simulink model "vehicle_suspension"  (R2016a)
settings: Solver=VariableStepAuto  SolverMode=SingleTasking  StartTime=0.0  StopTime=10.0  RelTol=1e-3
values from neighbouring files (symbols this model uses):
  Vmass = 2000    [vehicle_suspension_data.mat]
  wheeltrack = 1.5    [vehicle_suspension_data.mat]
  x_dist_pass1 = 0.6    [vehicle_suspension_data.mat]
  x_dist_pass2 = 1.1    [vehicle_suspension_data.mat]
  x_dist_pass3 = 0.6    [vehicle_suspension_data.mat]
  x_dist_pass4 = 1.1    [vehicle_suspension_data.mat]
  y_dist_pass1 = 1.4    [vehicle_suspension_data.mat]
  y_dist_pass2 = 1.4    [vehicle_suspension_data.mat]
  y_dist_pass3 = 2.2    [vehicle_suspension_data.mat]
  y_dist_pass4 = 2.2    [vehicle_suspension_data.mat]
settings Model: Creator=ADYPU-LAP-3  LastModifiedBy=AkashG_v13
settings DataIOCC: ReturnWorkspaceOutputs=on
settings DebuggingCC: SFUnexpectedBacktrackingDiag=error  SFNoUnconditionalDefaultTransitionDiag=error
settings SFSimCC: SimUseLocalCustomCode=on
settings RTWCC: RTWUseLocalCustomCode=on
settings GRTTargetCC: TargetLangStandard=C99 (ISO)  GeneratePreprocessorConditionals=Use local settings
settings ConfigComp: CovMetricSettings=dwe  CovHtmlReporting=off  CovSaveCumulativeToWorkspaceVar=off  CovSaveSingleToWorkspaceVar=off  CovExternalEMLEnable=on

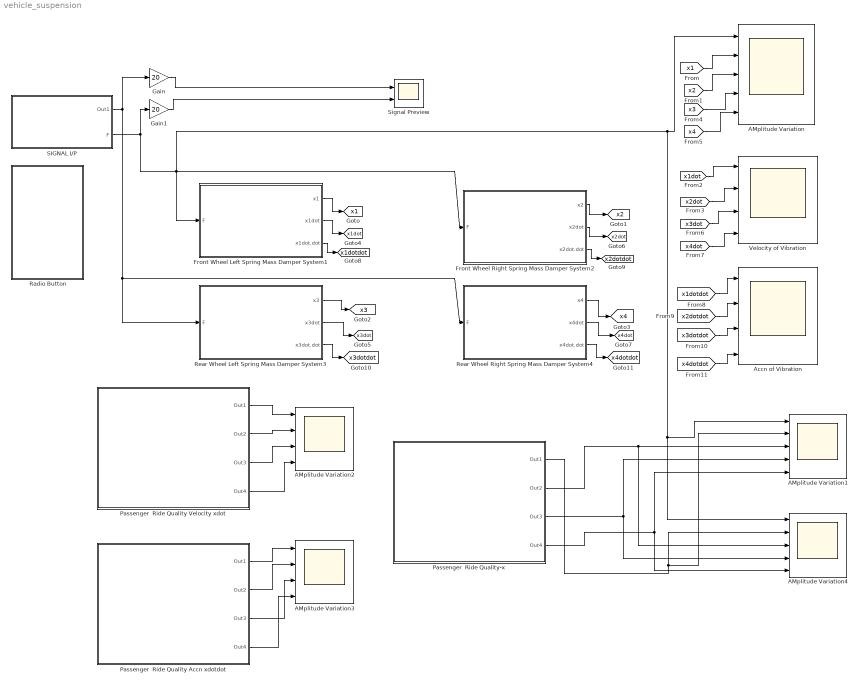
== system vehicle_suspension ==
  AMplitude Variation : Scope  NumInputPorts=5
  AMplitude Variation1 : Scope  NumInputPorts=5
  AMplitude Variation2 : Scope  NumInputPorts=4
  AMplitude Variation3 : Scope  NumInputPorts=4
  AMplitude Variation4 : Scope  NumInputPorts=5
  Accn of Vibration : Scope  NumInputPorts=4
  Front Wheel Left Spring Mass Damper System1 : Subsystem
  Front Wheel Right Spring Mass Damper System2 : Subsystem
  Gain : Gain  Gain=20
  Gain1 : Gain  Gain=20
  Passenger  Ride Quality Accn xdotdot : Subsystem
  Passenger  Ride Quality Velocity xdot : Subsystem
  Passenger  Ride Quality-x : Subsystem
  Radio Button : Subsystem  Description=Replaced Block  mask(Replaced Block){}
      mask help: This block has been replaced with an empty subsystem because it used functionality that is unavailable in Simulink R2016a.
      mask Display: fprintf('Replaced: %s\n','Dashboard Widget')
  Rear Wheel Left Spring Mass Damper System3 : Subsystem
  Rear Wheel Right Spring Mass Damper System4 : Subsystem
  SIGNAL I/P : Subsystem
  Signal Preview : Scope  NumInputPorts=2
  Velocity of Vibration : Scope  NumInputPorts=4
  tag scope: x1=global, x1dot=global, x1dotdot=global, x2=global, x2dot=global, x2dotdot=global, x3=global, x3dot=global, x3dotdot=global, x4=global, x4dot=global, x4dotdot=global
  wires:
  Front Wheel Left Spring Mass Damper System1/1(x1) -> [x1]
  Front Wheel Right Spring Mass Damper System2/1(x2) -> [x2]
  [x1] -> AMplitude Variation/2
  [x2] -> AMplitude Variation/3
  Rear Wheel Left Spring Mass Damper System3/1(x3) -> [x3]
  [x3] -> AMplitude Variation/4
  [x4] -> AMplitude Variation/5
  Rear Wheel Right Spring Mass Damper System4/1(x4) -> [x4]
  Passenger  Ride Quality-x/1(Out1) -> AMplitude Variation4/2, AMplitude Variation1/2
  Passenger  Ride Quality-x/3(Out3) -> AMplitude Variation1/4, AMplitude Variation4/4
  Passenger  Ride Quality-x/4(Out4) -> AMplitude Variation1/5, AMplitude Variation4/5
  Passenger  Ride Quality Velocity xdot/1(Out1) -> AMplitude Variation2/1
  Passenger  Ride Quality Velocity xdot/2(Out2) -> AMplitude Variation2/2
  Passenger  Ride Quality Velocity xdot/3(Out3) -> AMplitude Variation2/3
  Passenger  Ride Quality Velocity xdot/4(Out4) -> AMplitude Variation2/4
  Passenger  Ride Quality Accn xdotdot/1(Out1) -> AMplitude Variation3/1
  Passenger  Ride Quality Accn xdotdot/2(Out2) -> AMplitude Variation3/2
  Passenger  Ride Quality Accn xdotdot/3(Out3) -> AMplitude Variation3/3
  Passenger  Ride Quality Accn xdotdot/4(Out4) -> AMplitude Variation3/4
  Front Wheel Left Spring Mass Damper System1/2(x1dot) -> [x1dot]
  [x1dot] -> Velocity of Vibration/1
  Front Wheel Right Spring Mass Damper System2/2(x2dot) -> [x2dot]
  [x2dot] -> Velocity of Vibration/2
  Rear Wheel Left Spring Mass Damper System3/2(x3dot) -> [x3dot]
  [x3dot] -> Velocity of Vibration/3
  [x4dot] -> Velocity of Vibration/4
  Front Wheel Left Spring Mass Damper System1/3(x1dot.dot) -> [x1dotdot]
  Front Wheel Right Spring Mass Damper System2/3(x2dot.dot) -> [x2dotdot]
  Rear Wheel Left Spring Mass Damper System3/3(x3dot.dot) -> [x3dotdot]
  Rear Wheel Right Spring Mass Damper System4/2(x4dot) -> [x4dot]
  Rear Wheel Right Spring Mass Damper System4/3(x4dot.dot) -> [x4dotdot]
  [x1dotdot] -> Accn of Vibration/1
  [x2dotdot] -> Accn of Vibration/2
  [x3dotdot] -> Accn of Vibration/3
  [x4dotdot] -> Accn of Vibration/4
  Gain/1 -> Signal Preview/1
  Gain1/1 -> Signal Preview/2
  Passenger  Ride Quality-x/2(Out2) -> AMplitude Variation4/3, AMplitude Variation1/3
  SIGNAL I/P/2(F) -> Gain1/1, Front Wheel Left Spring Mass Damper System1/1(F), Front Wheel Right Spring Mass Damper System2/1(F), AMplitude Variation4/1, AMplitude Variation1/1, AMplitude Variation/1
  SIGNAL I/P/1(Out1) -> Rear Wheel Right Spring Mass Damper System4/1(F), Rear Wheel Left Spring Mass Damper System3/1(F), Gain/1

== system vehicle_suspension/Front Wheel Left Spring Mass Damper System1 ==
  F : Inport
  Add : Sum  Inputs=+---
  C-damping Coefficient : Gain  Gain=0.2
  Integrator : Integrator
  Integrator1 : Integrator
  Integrator2 : Integrator
  Mass-M1 : Gain  Gain=Vmass*(1.6/4)*0.5
  Spring Stiffness -K1 : Gain  Gain=2
  Spring Stifness K2 : Gain  Gain=5
  x1 : Outport
  x1dot : Outport  Port=2
  x1dot.dot : Outport  Port=3
  wires:
  C-damping Coefficient/1 -> Add/4  "C dx/dt"
  Integrator1/1 -> C-damping Coefficient/1, Integrator/1
  Spring Stiffness -K1/1 -> Add/2  "K1x"
  Integrator/1 -> x1/1, Spring Stifness K2/1, Spring Stiffness -K1/1  "x"
  Mass-M1/1 -> Integrator1/1  "M dx2/dt2"
  Spring Stifness K2/1 -> Add/3  "K2x"
  Add/1 -> Integrator2/1, x1dot.dot/1, Mass-M1/1  "d2x/dt2"
  F/1 -> Add/1
  Integrator2/1 -> x1dot/1

== system vehicle_suspension/Front Wheel Right Spring Mass Damper System2 ==
  F : Inport
  Add : Sum  Inputs=+---
  C-damping Coefficient : Gain  Gain=0.2
  Integrator : Integrator
  Integrator1 : Integrator
  Integrator2 : Integrator
  Mass-M1 : Gain  Gain=Vmass*(1.6/4)*0.5
  Spring Stiffness -K1 : Gain  Gain=2
  Spring Stifness K2 : Gain  Gain=5
  x2 : Outport
  x2dot : Outport  Port=2
  x2dot.dot : Outport  Port=3
  wires:
  Integrator2/1 -> x2dot/1
  F/1 -> Add/1
  Add/1 -> Mass-M1/1, x2dot.dot/1, Integrator2/1  "d2x/dt2"
  Spring Stifness K2/1 -> Add/3  "K2x"
  Mass-M1/1 -> Integrator1/1  "M dx2/dt2"
  Integrator/1 -> Spring Stiffness -K1/1, Spring Stifness K2/1, x2/1  "x2"
  Spring Stiffness -K1/1 -> Add/2  "K1x"
  Integrator1/1 -> Integrator/1, C-damping Coefficient/1
  C-damping Coefficient/1 -> Add/4  "C dx/dt"

== system vehicle_suspension/Passenger  Ride Quality Accn xdotdot ==
  Passenger 1 Ride Eval  x1 : Subsystem
  Passenger 2 Ride Eval  x2 : Subsystem
  Passenger 3 Ride Eval  x3 : Subsystem
  Passenger 4 Ride Eval  x4 : Subsystem
  Out1 : Outport
  Out2 : Outport  Port=2
  Out3 : Outport  Port=3
  Out4 : Outport  Port=4
  wires:
  Passenger 2 Ride Eval  x2/1(Out1) -> Out2/1
  Passenger 3 Ride Eval  x3/1(Out1) -> Out3/1
  Passenger 4 Ride Eval  x4/1(Out1) -> Out4/1
  Passenger 1 Ride Eval  x1/1(Out1) -> Out1/1

== system vehicle_suspension/Passenger  Ride Quality Velocity xdot ==
  Passenger 1 Ride Eval  x1 : Subsystem
  Passenger 2 Ride Eval  x2 : Subsystem
  Passenger 3 Ride Eval  x3 : Subsystem
  Passenger 4 Ride Eval  x4 : Subsystem
  Out1 : Outport
  Out2 : Outport  Port=2
  Out3 : Outport  Port=3
  Out4 : Outport  Port=4
  wires:
  Passenger 1 Ride Eval  x1/1(Out1) -> Out1/1
  Passenger 4 Ride Eval  x4/1(Out1) -> Out4/1
  Passenger 3 Ride Eval  x3/1(Out1) -> Out3/1
  Passenger 2 Ride Eval  x2/1(Out1) -> Out2/1

== system vehicle_suspension/Passenger  Ride Quality-x ==
  Passenger 1 Ride Eval  x1 : Subsystem
  Passenger 2 Ride Eval  x2 : Subsystem
  Passenger 3 Ride Eval  x3 : Subsystem
  Passenger 4 Ride Eval  x4 : Subsystem
  Out1 : Outport
  Out2 : Outport  Port=2
  Out3 : Outport  Port=3
  Out4 : Outport  Port=4
  wires:
  Passenger 2 Ride Eval  x2/1(Out1) -> Out2/1
  Passenger 3 Ride Eval  x3/1(Out1) -> Out3/1
  Passenger 4 Ride Eval  x4/1(Out1) -> Out4/1
  Passenger 1 Ride Eval  x1/1(Out1) -> Out1/1

== system vehicle_suspension/Radio Button ==

== system vehicle_suspension/Rear Wheel Left Spring Mass Damper System3 ==
  F : Inport
  Add : Sum  Inputs=+---
  C-damping Coefficient : Gain  Gain=0.2
  Integrator : Integrator
  Integrator1 : Integrator
  Integrator2 : Integrator
  Mass-M1 : Gain  Gain=Vmass*(1.6/4)*0.5
  Spring Stiffness -K1 : Gain  Gain=2
  Spring Stifness K2 : Gain  Gain=5
  x3 : Outport
  x3dot : Outport  Port=2
  x3dot.dot : Outport  Port=3
  wires:
  C-damping Coefficient/1 -> Add/4  "C dx/dt"
  Integrator1/1 -> C-damping Coefficient/1, Integrator/1
  Spring Stiffness -K1/1 -> Add/2  "K1x"
  Integrator/1 -> x3/1, Spring Stifness K2/1, Spring Stiffness -K1/1  "x3"
  Mass-M1/1 -> Integrator1/1  "M dx2/dt2"
  Spring Stifness K2/1 -> Add/3  "K2x"
  Add/1 -> Integrator2/1, x3dot.dot/1, Mass-M1/1  "d2x/dt2"
  F/1 -> Add/1
  Integrator2/1 -> x3dot/1

== system vehicle_suspension/Rear Wheel Right Spring Mass Damper System4 ==
  F : Inport
  Add : Sum  Inputs=+---
  C-damping Coefficient : Gain  Gain=0.2
  Integrator : Integrator
  Integrator1 : Integrator
  Integrator2 : Integrator
  Mass-M1 : Gain  Gain=Vmass*(1.6/4)*0.5
  Spring Stiffness -K1 : Gain  Gain=2
  Spring Stifness K2 : Gain  Gain=5
  x4 : Outport
  x4dot : Outport  Port=2
  x4dot.dot : Outport  Port=3
  wires:
  Integrator2/1 -> x4dot/1
  F/1 -> Add/1
  Add/1 -> Mass-M1/1, x4dot.dot/1, Integrator2/1  "d2x/dt2"
  Spring Stifness K2/1 -> Add/3  "K2x"
  Mass-M1/1 -> Integrator1/1  "M dx2/dt2"
  Integrator/1 -> Spring Stiffness -K1/1, Spring Stifness K2/1, x4/1  "x4"
  Spring Stiffness -K1/1 -> Add/2  "K1x"
  Integrator1/1 -> Integrator/1, C-damping Coefficient/1
  C-damping Coefficient/1 -> Add/4  "C dx/dt"

== system vehicle_suspension/SIGNAL I//P ==
  " " : Trigonometry  Operator=cos
  Add : Sum  Inputs=+-
  Clock : Clock
      settings: Decimation=20
  Constant1 : Constant  Value=2
  Constant2 : Constant  Value=2
  Product : Product
  Product1 : Product
  Sin : Trigonometry  Operator=cos
  Out1 : Outport
  F : Outport  Port=2
  wires:
  Constant1/1 -> Product1/1, Product/1
  Constant2/1 -> Add/2
  Add/1 -> " "/1
  " "/1 -> F/1  "F"
  Product1/1 -> Add/1
  Product/1 -> Sin/1
  Clock/1 -> Product1/2, Product/2
  Sin/1 -> Out1/1

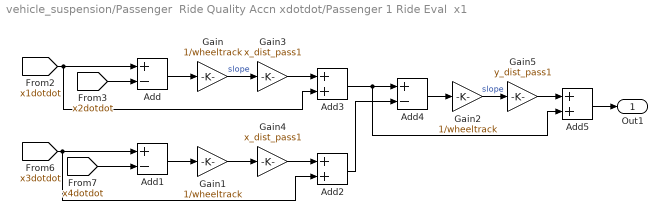
== system vehicle_suspension/Passenger  Ride Quality Accn xdotdot/Passenger 1 Ride Eval  x1 ==
  Add : Sum  Inputs=+-
  Add1 : Sum  Inputs=+-
  Add2 : Sum
  Add3 : Sum
  Add4 : Sum  Inputs=+-
  Add5 : Sum
  Gain : Gain  Gain=1/wheeltrack
  Gain1 : Gain  Gain=1/wheeltrack
  Gain2 : Gain  Gain=1/wheeltrack
  Gain3 : Gain  Gain=x_dist_pass1
  Gain4 : Gain  Gain=x_dist_pass1
  Gain5 : Gain  Gain=y_dist_pass1
  Out1 : Outport
  wires:
  Gain1/1 -> Gain4/1
  [x2dotdot] -> Add/2
  Gain2/1 -> Gain5/1  "slope"
  Gain/1 -> Gain3/1  "slope"
  [x4dotdot] -> Add1/2
  Add1/1 -> Gain1/1
  [x1dotdot] -> Add3/2, Add/1
  Add/1 -> Gain/1
  Gain3/1 -> Add3/1
  Gain4/1 -> Add2/1
  [x3dotdot] -> Add2/2, Add1/1
  Add3/1 -> Add5/2, Add4/1
  Add2/1 -> Add4/2
  Add4/1 -> Gain2/1
  Gain5/1 -> Add5/1
  Add5/1 -> Out1/1

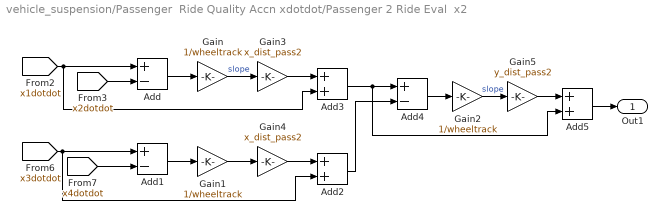
== system vehicle_suspension/Passenger  Ride Quality Accn xdotdot/Passenger 2 Ride Eval  x2 ==
  Add : Sum  Inputs=+-
  Add1 : Sum  Inputs=+-
  Add2 : Sum
  Add3 : Sum
  Add4 : Sum  Inputs=+-
  Add5 : Sum
  Gain : Gain  Gain=1/wheeltrack
  Gain1 : Gain  Gain=1/wheeltrack
  Gain2 : Gain  Gain=1/wheeltrack
  Gain3 : Gain  Gain=x_dist_pass2
  Gain4 : Gain  Gain=x_dist_pass2
  Gain5 : Gain  Gain=y_dist_pass2
  Out1 : Outport
  wires:
  Add5/1 -> Out1/1
  Gain5/1 -> Add5/1
  Add4/1 -> Gain2/1
  Add2/1 -> Add4/2
  Add3/1 -> Add4/1, Add5/2
  [x3dotdot] -> Add1/1, Add2/2
  Gain4/1 -> Add2/1
  Gain3/1 -> Add3/1
  Add/1 -> Gain/1
  [x1dotdot] -> Add/1, Add3/2
  Add1/1 -> Gain1/1
  [x4dotdot] -> Add1/2
  Gain/1 -> Gain3/1  "slope"
  Gain2/1 -> Gain5/1  "slope"
  [x2dotdot] -> Add/2
  Gain1/1 -> Gain4/1

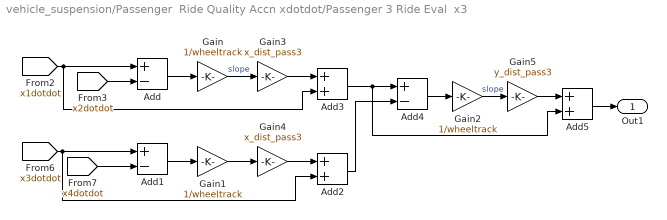
== system vehicle_suspension/Passenger  Ride Quality Accn xdotdot/Passenger 3 Ride Eval  x3 ==
  Add : Sum  Inputs=+-
  Add1 : Sum  Inputs=+-
  Add2 : Sum
  Add3 : Sum
  Add4 : Sum  Inputs=+-
  Add5 : Sum
  Gain : Gain  Gain=1/wheeltrack
  Gain1 : Gain  Gain=1/wheeltrack
  Gain2 : Gain  Gain=1/wheeltrack
  Gain3 : Gain  Gain=x_dist_pass3
  Gain4 : Gain  Gain=x_dist_pass3
  Gain5 : Gain  Gain=y_dist_pass3
  Out1 : Outport
  wires:
  Gain1/1 -> Gain4/1
  [x2dotdot] -> Add/2
  Gain2/1 -> Gain5/1  "slope"
  Gain/1 -> Gain3/1  "slope"
  [x4dotdot] -> Add1/2
  Add1/1 -> Gain1/1
  [x1dotdot] -> Add3/2, Add/1
  Add/1 -> Gain/1
  Gain3/1 -> Add3/1
  Gain4/1 -> Add2/1
  [x3dotdot] -> Add2/2, Add1/1
  Add3/1 -> Add5/2, Add4/1
  Add2/1 -> Add4/2
  Add4/1 -> Gain2/1
  Gain5/1 -> Add5/1
  Add5/1 -> Out1/1

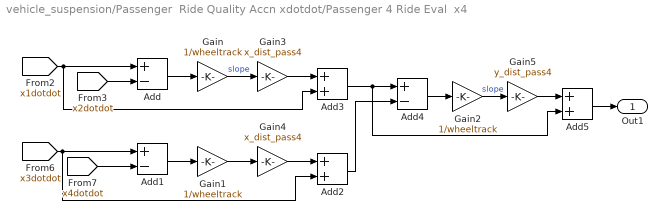
== system vehicle_suspension/Passenger  Ride Quality Accn xdotdot/Passenger 4 Ride Eval  x4 ==
  Add : Sum  Inputs=+-
  Add1 : Sum  Inputs=+-
  Add2 : Sum
  Add3 : Sum
  Add4 : Sum  Inputs=+-
  Add5 : Sum
  Gain : Gain  Gain=1/wheeltrack
  Gain1 : Gain  Gain=1/wheeltrack
  Gain2 : Gain  Gain=1/wheeltrack
  Gain3 : Gain  Gain=x_dist_pass4
  Gain4 : Gain  Gain=x_dist_pass4
  Gain5 : Gain  Gain=y_dist_pass4
  Out1 : Outport
  wires:
  Add5/1 -> Out1/1
  Gain5/1 -> Add5/1
  Add4/1 -> Gain2/1
  Add2/1 -> Add4/2
  Add3/1 -> Add4/1, Add5/2
  [x3dotdot] -> Add1/1, Add2/2
  Gain4/1 -> Add2/1
  Gain3/1 -> Add3/1
  Add/1 -> Gain/1
  [x1dotdot] -> Add/1, Add3/2
  Add1/1 -> Gain1/1
  [x4dotdot] -> Add1/2
  Gain/1 -> Gain3/1  "slope"
  Gain2/1 -> Gain5/1  "slope"
  [x2dotdot] -> Add/2
  Gain1/1 -> Gain4/1

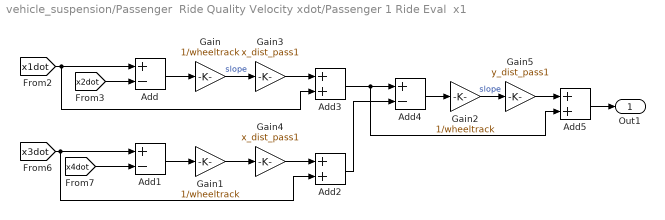
== system vehicle_suspension/Passenger  Ride Quality Velocity xdot/Passenger 1 Ride Eval  x1 ==
  Add : Sum  Inputs=+-
  Add1 : Sum  Inputs=+-
  Add2 : Sum
  Add3 : Sum
  Add4 : Sum  Inputs=+-
  Add5 : Sum
  Gain : Gain  Gain=1/wheeltrack
  Gain1 : Gain  Gain=1/wheeltrack
  Gain2 : Gain  Gain=1/wheeltrack
  Gain3 : Gain  Gain=x_dist_pass1
  Gain4 : Gain  Gain=x_dist_pass1
  Gain5 : Gain  Gain=y_dist_pass1
  Out1 : Outport
  wires:
  Add5/1 -> Out1/1
  Gain5/1 -> Add5/1
  Add4/1 -> Gain2/1
  Add2/1 -> Add4/2
  Add3/1 -> Add4/1, Add5/2
  [x3dot] -> Add1/1, Add2/2
  Gain4/1 -> Add2/1
  Gain3/1 -> Add3/1
  Add/1 -> Gain/1
  [x1dot] -> Add/1, Add3/2
  Add1/1 -> Gain1/1
  [x4dot] -> Add1/2
  Gain/1 -> Gain3/1  "slope"
  Gain2/1 -> Gain5/1  "slope"
  [x2dot] -> Add/2
  Gain1/1 -> Gain4/1

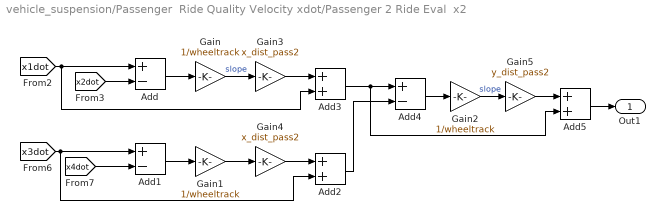
== system vehicle_suspension/Passenger  Ride Quality Velocity xdot/Passenger 2 Ride Eval  x2 ==
  Add : Sum  Inputs=+-
  Add1 : Sum  Inputs=+-
  Add2 : Sum
  Add3 : Sum
  Add4 : Sum  Inputs=+-
  Add5 : Sum
  Gain : Gain  Gain=1/wheeltrack
  Gain1 : Gain  Gain=1/wheeltrack
  Gain2 : Gain  Gain=1/wheeltrack
  Gain3 : Gain  Gain=x_dist_pass2
  Gain4 : Gain  Gain=x_dist_pass2
  Gain5 : Gain  Gain=y_dist_pass2
  Out1 : Outport
  wires:
  Gain1/1 -> Gain4/1
  [x2dot] -> Add/2
  Gain2/1 -> Gain5/1  "slope"
  Gain/1 -> Gain3/1  "slope"
  [x4dot] -> Add1/2
  Add1/1 -> Gain1/1
  [x1dot] -> Add3/2, Add/1
  Add/1 -> Gain/1
  Gain3/1 -> Add3/1
  Gain4/1 -> Add2/1
  [x3dot] -> Add2/2, Add1/1
  Add3/1 -> Add5/2, Add4/1
  Add2/1 -> Add4/2
  Add4/1 -> Gain2/1
  Gain5/1 -> Add5/1
  Add5/1 -> Out1/1

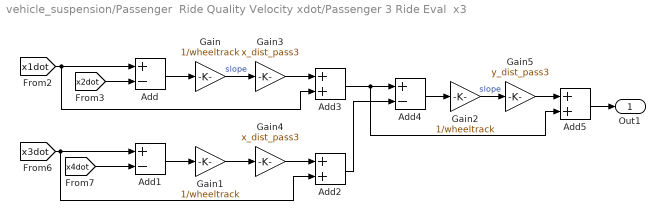
== system vehicle_suspension/Passenger  Ride Quality Velocity xdot/Passenger 3 Ride Eval  x3 ==
  Add : Sum  Inputs=+-
  Add1 : Sum  Inputs=+-
  Add2 : Sum
  Add3 : Sum
  Add4 : Sum  Inputs=+-
  Add5 : Sum
  Gain : Gain  Gain=1/wheeltrack
  Gain1 : Gain  Gain=1/wheeltrack
  Gain2 : Gain  Gain=1/wheeltrack
  Gain3 : Gain  Gain=x_dist_pass3
  Gain4 : Gain  Gain=x_dist_pass3
  Gain5 : Gain  Gain=y_dist_pass3
  Out1 : Outport
  wires:
  Add5/1 -> Out1/1
  Gain5/1 -> Add5/1
  Add4/1 -> Gain2/1
  Add2/1 -> Add4/2
  Add3/1 -> Add4/1, Add5/2
  [x3dot] -> Add1/1, Add2/2
  Gain4/1 -> Add2/1
  Gain3/1 -> Add3/1
  Add/1 -> Gain/1
  [x1dot] -> Add/1, Add3/2
  Add1/1 -> Gain1/1
  [x4dot] -> Add1/2
  Gain/1 -> Gain3/1  "slope"
  Gain2/1 -> Gain5/1  "slope"
  [x2dot] -> Add/2
  Gain1/1 -> Gain4/1

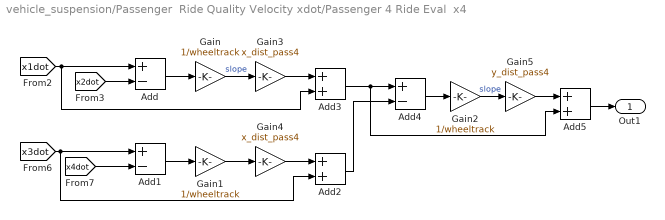
== system vehicle_suspension/Passenger  Ride Quality Velocity xdot/Passenger 4 Ride Eval  x4 ==
  Add : Sum  Inputs=+-
  Add1 : Sum  Inputs=+-
  Add2 : Sum
  Add3 : Sum
  Add4 : Sum  Inputs=+-
  Add5 : Sum
  Gain : Gain  Gain=1/wheeltrack
  Gain1 : Gain  Gain=1/wheeltrack
  Gain2 : Gain  Gain=1/wheeltrack
  Gain3 : Gain  Gain=x_dist_pass4
  Gain4 : Gain  Gain=x_dist_pass4
  Gain5 : Gain  Gain=y_dist_pass4
  Out1 : Outport
  wires:
  Gain1/1 -> Gain4/1
  [x2dot] -> Add/2
  Gain2/1 -> Gain5/1  "slope"
  Gain/1 -> Gain3/1  "slope"
  [x4dot] -> Add1/2
  Add1/1 -> Gain1/1
  [x1dot] -> Add3/2, Add/1
  Add/1 -> Gain/1
  Gain3/1 -> Add3/1
  Gain4/1 -> Add2/1
  [x3dot] -> Add2/2, Add1/1
  Add3/1 -> Add5/2, Add4/1
  Add2/1 -> Add4/2
  Add4/1 -> Gain2/1
  Gain5/1 -> Add5/1
  Add5/1 -> Out1/1

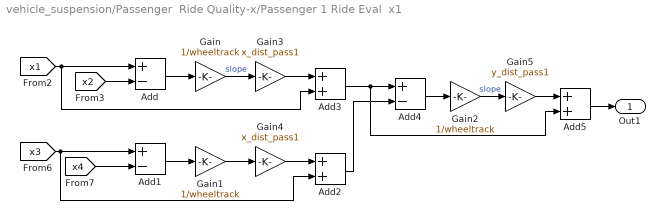
== system vehicle_suspension/Passenger  Ride Quality-x/Passenger 1 Ride Eval  x1 ==
  Add : Sum  Inputs=+-
  Add1 : Sum  Inputs=+-
  Add2 : Sum
  Add3 : Sum
  Add4 : Sum  Inputs=+-
  Add5 : Sum
  Gain : Gain  Gain=1/wheeltrack
  Gain1 : Gain  Gain=1/wheeltrack
  Gain2 : Gain  Gain=1/wheeltrack
  Gain3 : Gain  Gain=x_dist_pass1
  Gain4 : Gain  Gain=x_dist_pass1
  Gain5 : Gain  Gain=y_dist_pass1
  Out1 : Outport
  wires:
  Gain1/1 -> Gain4/1
  [x2] -> Add/2
  Gain2/1 -> Gain5/1  "slope"
  Gain/1 -> Gain3/1  "slope"
  [x4] -> Add1/2
  Add1/1 -> Gain1/1
  [x1] -> Add3/2, Add/1
  Add/1 -> Gain/1
  Gain3/1 -> Add3/1
  Gain4/1 -> Add2/1
  [x3] -> Add2/2, Add1/1
  Add3/1 -> Add5/2, Add4/1
  Add2/1 -> Add4/2
  Add4/1 -> Gain2/1
  Gain5/1 -> Add5/1
  Add5/1 -> Out1/1

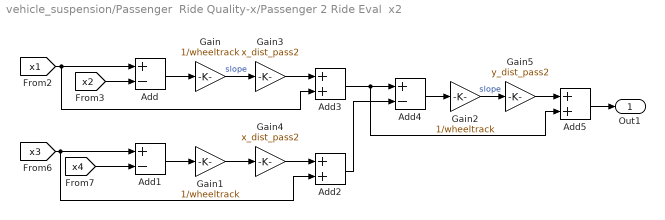
== system vehicle_suspension/Passenger  Ride Quality-x/Passenger 2 Ride Eval  x2 ==
  Add : Sum  Inputs=+-
  Add1 : Sum  Inputs=+-
  Add2 : Sum
  Add3 : Sum
  Add4 : Sum  Inputs=+-
  Add5 : Sum
  Gain : Gain  Gain=1/wheeltrack
  Gain1 : Gain  Gain=1/wheeltrack
  Gain2 : Gain  Gain=1/wheeltrack
  Gain3 : Gain  Gain=x_dist_pass2
  Gain4 : Gain  Gain=x_dist_pass2
  Gain5 : Gain  Gain=y_dist_pass2
  Out1 : Outport
  wires:
  Add5/1 -> Out1/1
  Gain5/1 -> Add5/1
  Add4/1 -> Gain2/1
  Add2/1 -> Add4/2
  Add3/1 -> Add4/1, Add5/2
  [x3] -> Add1/1, Add2/2
  Gain4/1 -> Add2/1
  Gain3/1 -> Add3/1
  Add/1 -> Gain/1
  [x1] -> Add/1, Add3/2
  Add1/1 -> Gain1/1
  [x4] -> Add1/2
  Gain/1 -> Gain3/1  "slope"
  Gain2/1 -> Gain5/1  "slope"
  [x2] -> Add/2
  Gain1/1 -> Gain4/1

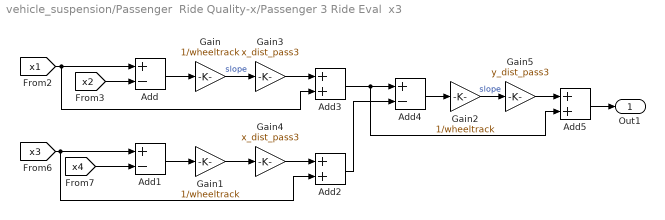
== system vehicle_suspension/Passenger  Ride Quality-x/Passenger 3 Ride Eval  x3 ==
  Add : Sum  Inputs=+-
  Add1 : Sum  Inputs=+-
  Add2 : Sum
  Add3 : Sum
  Add4 : Sum  Inputs=+-
  Add5 : Sum
  Gain : Gain  Gain=1/wheeltrack
  Gain1 : Gain  Gain=1/wheeltrack
  Gain2 : Gain  Gain=1/wheeltrack
  Gain3 : Gain  Gain=x_dist_pass3
  Gain4 : Gain  Gain=x_dist_pass3
  Gain5 : Gain  Gain=y_dist_pass3
  Out1 : Outport
  wires:
  Gain1/1 -> Gain4/1
  [x2] -> Add/2
  Gain2/1 -> Gain5/1  "slope"
  Gain/1 -> Gain3/1  "slope"
  [x4] -> Add1/2
  Add1/1 -> Gain1/1
  [x1] -> Add3/2, Add/1
  Add/1 -> Gain/1
  Gain3/1 -> Add3/1
  Gain4/1 -> Add2/1
  [x3] -> Add2/2, Add1/1
  Add3/1 -> Add5/2, Add4/1
  Add2/1 -> Add4/2
  Add4/1 -> Gain2/1
  Gain5/1 -> Add5/1
  Add5/1 -> Out1/1

== system vehicle_suspension/Passenger  Ride Quality-x/Passenger 4 Ride Eval  x4 ==
  Add : Sum  Inputs=+-
  Add1 : Sum  Inputs=+-
  Add2 : Sum
  Add3 : Sum
  Add4 : Sum  Inputs=+-
  Add5 : Sum
  Gain : Gain  Gain=1/wheeltrack
  Gain1 : Gain  Gain=1/wheeltrack
  Gain2 : Gain  Gain=1/wheeltrack
  Gain3 : Gain  Gain=x_dist_pass4
  Gain4 : Gain  Gain=x_dist_pass4
  Gain5 : Gain  Gain=y_dist_pass4
  Out1 : Outport
  wires:
  Add5/1 -> Out1/1
  Gain5/1 -> Add5/1
  Add4/1 -> Gain2/1
  Add2/1 -> Add4/2
  Add3/1 -> Add4/1, Add5/2
  [x3] -> Add1/1, Add2/2
  Gain4/1 -> Add2/1
  Gain3/1 -> Add3/1
  Add/1 -> Gain/1
  [x1] -> Add/1, Add3/2
  Add1/1 -> Gain1/1
  [x4] -> Add1/2
  Gain/1 -> Gain3/1  "slope"
  Gain2/1 -> Gain5/1  "slope"
  [x2] -> Add/2
  Gain1/1 -> Gain4/1
